simulink model "MCSI_simulation_2024_using_pc_source_and_cuantized_signals"  (R2021a)
settings: Solver=VariableStepAuto  StartTime=0.0  StopTime=10/cfg.fl  RelTol=1e-3
undefined symbols (not defined in the file or in its folder): cfg
libraries: spsIdealSwitchLib x18, simulink x8, spsSeriesRLCBranchLib x8, spsCurrentMeasurementLib x6, spsMosfetLib x4, commutil2 x3, spsTriangleGeneratorLib x3, spsMeanLib x2, spsThreePhaseSeriesRLCBranchLib x2, spsThreePhaseVIMeasurementLib x2, spspowerguiLib x2, spsGroundLib x1
settings Model: Creator=Damian  LastModifiedBy=Damian

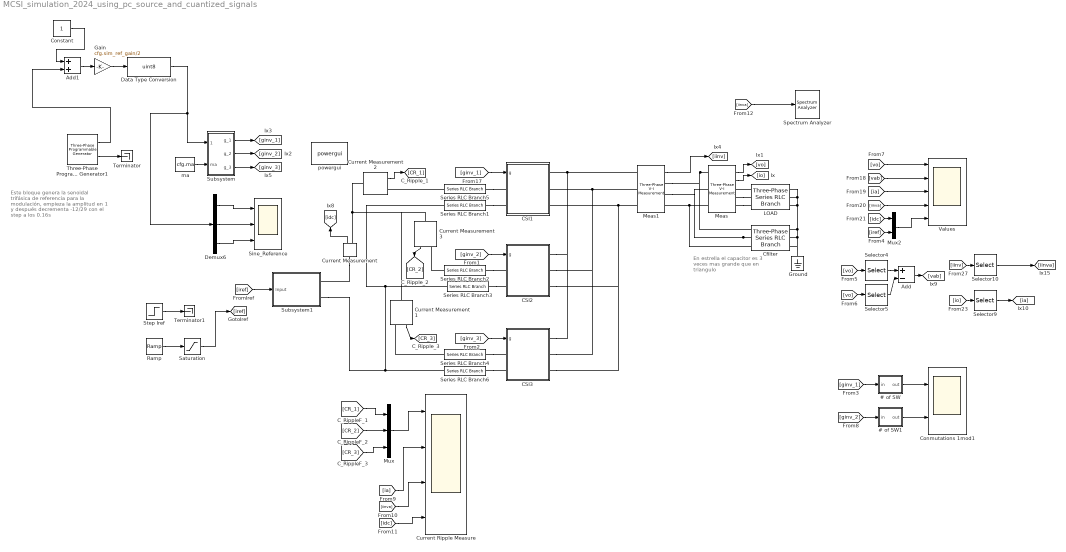
== system MCSI_simulation_2024_using_pc_source_and_cuantized_signals ==
  note: Este bloque genera la senoidal
      | trifásica de referencia para la
      | modulación, empieza la amplitud
      | en 1 y después decrementa -12/29
      | con el step a los 0.16s
  note: En estrella el capacitor
      | es 3 veces mas grande
      | que en triangulo
  # of SW : Subsystem
  # of SW1 : Subsystem
  Add : Sum  Inputs=+-
  Add1 : Sum
  CSI1 : Subsystem
  CSI2 : Subsystem
  CSI3 : Subsystem
  Cfilter : spsThreePhaseSeriesRLCBranchLib/Three-Phase Series RLC Branch  LConnTagsString=A|B|C  RConnTagsString=A|B|C  BranchType=C  Resistance=1  Inductance=cfg.c  Capacitance=cfg.c  Measurements=None
  Conmutations 1mod1 : Scope  NumInputPorts=2
  Constant : Constant
  Current Measurement{,1..3} (4 alike) : spsCurrentMeasurementLib/Current Measurement  PhasorSimulation=off  OutputType=Complex  PSBequivalent=0
  Current Ripple Measure : Scope  NumInputPorts=4
  Data Type Conversion : DataTypeConversion  OutDataTypeStr=uint8
  Demux6 : Demux  Outputs=3
  Gain : Gain  Gain=cfg.sim_ref_gain/2
  Ground : spsGroundLib/Ground  LConnTagsString=a
  LOAD : spsThreePhaseSeriesRLCBranchLib/Three-Phase Series RLC Branch  LConnTagsString=A|B|C  RConnTagsString=A|B|C  BranchType=RL  Resistance=cfg.r  Inductance=cfg.l  Capacitance=1e-6  Measurements=None
  Meas : spsThreePhaseVIMeasurementLib/Three-Phase V-I Measurement  VoltageMeasurement=phase-to-ground  SetLabelV=off  LabelV=Vabc  Vpu=off  VpuLL=off  CurrentMeasurement=yes  SetLabelI=off  LabelI=Iabc  Ipu=off  Pbase=100e6  Vbase=500e3  OutputType=Complex  PhasorSimulation=off  PSBequivalent=0
  Meas1 : spsThreePhaseVIMeasurementLib/Three-Phase V-I Measurement  VoltageMeasurement=no  SetLabelV=off  LabelV=Vabc  Vpu=off  VpuLL=off  CurrentMeasurement=yes  SetLabelI=off  LabelI=Iabc  Ipu=off  Pbase=100e6  Vbase=500e3  OutputType=Complex  PhasorSimulation=off  PSBequivalent=0
  Mux : Mux  Inputs=3
  Mux2 : Mux  Inputs=2
  Ramp : simulink/Sources/Ramp  slope=cfg.iref/cfg.cs_soft_start_time  start=0  InitialOutput=0
  Saturation : Saturate  UpperLimit=cfg.iref  LowerLimit=0
  Selector10 : Selector  InputPortWidth=3  IndexOptions=Index vector (dialog)  Indices=1  OutputSizes=1
  Selector4 : Selector  InputPortWidth=3  IndexOptions=Index vector (dialog)  Indices=1  OutputSizes=1
  Selector5 : Selector  InputPortWidth=3  IndexOptions=Index vector (dialog)  Indices=2  OutputSizes=1
  Selector9 : Selector  InputPortWidth=3  IndexOptions=Index vector (dialog)  Indices=1  OutputSizes=1
  Series RLC Branch{1..6} (6 alike) : spsSeriesRLCBranchLib/Series RLC Branch  LConnTagsString=__new0  RConnTagsString=__new0  BranchType=RL  Resistance=cfg.sharing_R  Inductance=cfg.sharing_L  SetiL0=off  InitialCurrent=0  Capacitance=1e-6  Setx0=off  InitialVoltage=0  Measurements=None
  Sine_Reference : Scope  NumInputPorts=3
  Spectrum Analyzer : SpectrumAnalyzer
  Step Iref : Step  Time=12/cfg.fl  Before=cfg.iref  After=0.6*cfg.iref  SampleTime=cfg.ts
  Subsystem : Subsystem
  Subsystem1 : Subsystem
  Terminator : Terminator
  Terminator1 : Terminator
  Three-Phase Programmable Generator1 : spsThreePhaseProgrammableGeneratorLib/Three-Phase Programmable Generator  Par_Vps=[0.9999,-30, cfg.fl]  VariationEntity=None  VariationType=Step  VariationStep=-12/29  VariationRate=10  VariationMag=0.3  VariationFreq=2  Par_Timing_Variation="[8/cfg.fl  10]"  SinglePhase=on  Yampli=[1 0.2 1.2 1.0]  Xtime=[0 0.1 0.15 0.2]  HarmonicGeneration=off  Par_HarmoA="[3  5  -25 0]"  Par_HarmoB="[5  10  35  2]"  Par_Timing_Harmo="[ 0.05  99]"  Ts=cfg.ts
      settings: SourceProductBaseCode=PS
  Values : Scope  NumInputPorts=5
  ma : Constant  Value=cfg.ma
  powergui : spspowerguiLib/powergui  Priority=1  SimulationMode=Discrete  SampleTime=cfg.ts  frequency=60  Iterations=50  frequencyindice=0  Pbase=100e6  ErrMax=1e-4  UnitsV=kV  UnitsW=MW  buscounter=0  FunctionMessages=off  echomessages=off  EnableUseOfTLC=off  CurrentSourceSwitches=off  DisableSnubberDevices=off  DisableRonSwitches=off  DisableVfSwitches=off  DisplayEquations=off  AutomaticDiscreteSolvers=off  SolverType=Backward Euler  Interpol=off  ExternalGateDelay=off  methode=off  Ts=0  x0status=blocks  SPID=off  SwTol=0  HookPort=off  NonlinearTolerance=1e-4  nMaxIteration=100  ContinueOnMaxIteration=off  RestoreLinks=warning  ResistiveCurrentMeasurement=off  Frange=[0:2:500]  Ylog=off  Xlog=on  ShowGrid=off  save=off  variable=ZData  structure=one_mod_model  ZoomFFT=off  StartTime=0.12  cycles=1  DisplayStyle=1  fundamental=50  FreqAxis=off  MaxFrequency=1000  frequencyindicesteady=1  RmsSteady=1  display=off
  wires:
  Current Measurement/1 -> [idc]
  ma/1 -> Subsystem/2(ma)
  Subsystem/1(g_1) -> [ginv_1]
  Three-Phase Programmable Generator1/2 -> Terminator/1
  Demux6/3 -> Sine_Reference/3
  Demux6/2 -> Sine_Reference/2
  Demux6/1 -> Sine_Reference/1
  [ginv_1] -> CSI1/1(g)
  Meas/1 -> [vo]
  Meas/2 -> [io]
  Meas1/1 -> [iinv]
  [iref] -> Mux2/2
  [idc] -> Mux2/1
  Mux2/1 -> Values/5
  [vo] -> Values/1
  [iinva] -> Values/4
  [ia] -> Values/3
  [vab] -> Values/2
  [vo] -> Selector4/1
  [vo] -> Selector5/1
  Selector4/1 -> Add/1
  Selector5/1 -> Add/2
  Add/1 -> [vab]
  [iinv] -> Selector10/1
  [io] -> Selector9/1
  Selector10/1 -> [iinva]
  Selector9/1 -> [ia]
  Subsystem/3(g_3) -> [ginv_3]
  Subsystem/2(g_2) -> [ginv_2]
  [ginv_2] -> CSI2/1(g)
  [ginv_3] -> CSI3/1(g)
  [ginv_1] -> # of SW/1(in)
  # of SW/1(out) -> Conmutations 1mod1/1
  # of SW1/1(out) -> Conmutations 1mod1/2
  [ginv_2] -> # of SW1/1(in)
  Saturation/1 -> [iref]
  Ramp/1 -> Saturation/1
  Step Iref/1 -> Terminator1/1
  Current Measurement2/1 -> [CR_1]
  Current Measurement3/1 -> [CR_2]
  Current Measurement1/1 -> [CR_3]
  [ia] -> Current Ripple Measure/2
  [iinva] -> Current Ripple Measure/3
  [idc] -> Current Ripple Measure/4
  [CR_1] -> Mux/1
  [CR_2] -> Mux/2
  [CR_3] -> Mux/3
  Mux/1 -> Current Ripple Measure/1
  [iref] -> Subsystem1/1(Input)
  Constant/1 -> Add1/1
  Gain/1 -> Data Type Conversion/1
  Add1/1 -> Gain/1
  Three-Phase Programmable Generator1/1 -> Add1/2
  Data Type Conversion/1 -> Demux6/1, Subsystem/1(Vabc)
  [iinva] -> Spectrum Analyzer/1
  connections:
  Current Measurement/LConn1 -- Subsystem1/RConn1
  Meas/LConn3 -- Cfilter/LConn3 -- Meas1/RConn3
  Meas/LConn1 -- Meas1/RConn1 -- Cfilter/LConn1
  LOAD/RConn2 -- LOAD/RConn1 -- LOAD/RConn3 -- Cfilter/RConn1 -- Cfilter/RConn2 -- Cfilter/RConn3 -- Ground/LConn1
  Cfilter/LConn2 -- Meas1/RConn2 -- Meas/LConn2
  LOAD/LConn1 -- Meas/RConn1
  Meas/RConn2 -- LOAD/LConn2
  Meas/RConn3 -- LOAD/LConn3
  Meas1/LConn1 -- CSI3/RConn1 -- CSI2/RConn1 -- CSI1/RConn1
  Meas1/LConn2 -- CSI3/RConn2 -- CSI2/RConn2 -- CSI1/RConn2
  Meas1/LConn3 -- CSI3/RConn3 -- CSI2/RConn3 -- CSI1/RConn3
  Series RLC Branch1/RConn1 -- CSI1/LConn2
  Series RLC Branch5/RConn1 -- CSI1/LConn1
  Series RLC Branch2/RConn1 -- CSI2/LConn1
  Series RLC Branch3/RConn1 -- CSI2/LConn2
  Series RLC Branch4/RConn1 -- CSI3/LConn1
  Series RLC Branch6/RConn1 -- CSI3/LConn2
  Subsystem1/RConn2 -- Series RLC Branch6/LConn1 -- Series RLC Branch3/LConn1 -- Series RLC Branch1/LConn1
  Series RLC Branch2/LConn1 -- Current Measurement3/RConn1
  Current Measurement2/LConn1 -- Current Measurement3/LConn1 -- Current Measurement1/LConn1 -- Current Measurement/RConn1
  Series RLC Branch4/LConn1 -- Current Measurement1/RConn1
  Series RLC Branch5/LConn1 -- Current Measurement2/RConn1

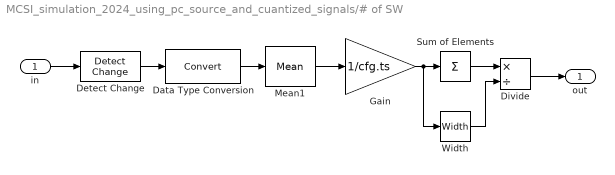
== system MCSI_simulation_2024_using_pc_source_and_cuantized_signals/# of SW ==
  in : Inport
  Data Type Conversion : DataTypeConversion
  Detect Change : simulink/Logic and Bit Operations/Detect Change  vinit=0  OutDataTypeStr=boolean
  Divide : Product  Inputs=*/
  Gain : Gain  Gain=1/cfg.ts
  Mean1 : spsMeanLib/Mean  Freq=cfg.fl  Vinit=0  Ts=cfg.ts
  Sum of Elements : Sum  Inputs=+
  Width : Width
  out : Outport
  wires:
  Detect Change/1 -> Data Type Conversion/1
  Mean1/1 -> Gain/1
  Data Type Conversion/1 -> Mean1/1
  in/1 -> Detect Change/1
  Gain/1 -> Width/1, Sum of Elements/1
  Sum of Elements/1 -> Divide/1
  Width/1 -> Divide/2
  Divide/1 -> out/1

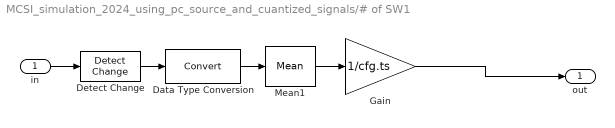
== system MCSI_simulation_2024_using_pc_source_and_cuantized_signals/# of SW1 ==
  in : Inport
  Data Type Conversion : DataTypeConversion
  Detect Change : simulink/Logic and Bit Operations/Detect Change  vinit=0  OutDataTypeStr=boolean
  Gain : Gain  Gain=1/cfg.ts
  Mean1 : spsMeanLib/Mean  Freq=cfg.fl  Vinit=0  Ts=cfg.ts
  out : Outport
  wires:
  Detect Change/1 -> Data Type Conversion/1
  Mean1/1 -> Gain/1
  Data Type Conversion/1 -> Mean1/1
  in/1 -> Detect Change/1
  Gain/1 -> out/1

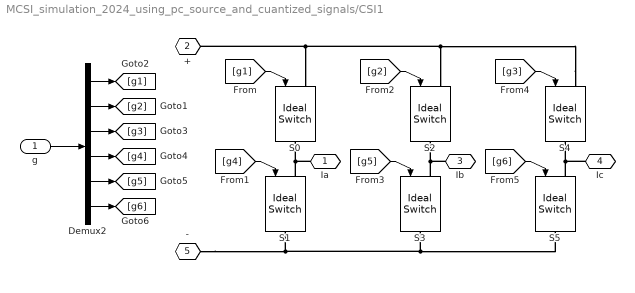
== system MCSI_simulation_2024_using_pc_source_and_cuantized_signals/CSI1 ==
  g : Inport
  Demux2 : Demux  Outputs=6
  S{0..5} (6 alike) : spsIdealSwitchLib/Ideal Switch  Ron=cfg.switch.Ron  Lon=0  IC=0  Rs=cfg.switch.snubber_Rs  Cs=cfg.switch.snubber_Cs  Measurements=off
  Ia : PMIOPort  Side=Right
  + : PMIOPort  Port=2  Side=Left
  Ib : PMIOPort  Port=3  Side=Right
  Ic : PMIOPort  Port=4  Side=Right
  - : PMIOPort  Port=5  Side=Left
  wires:
  Demux2/1 -> [g1]
  Demux2/4 -> [g4]
  g/1 -> Demux2/1
  [g4] -> S1/1
  [g2] -> S2/1
  [g5] -> S3/1
  Demux2/5 -> [g5]
  [g3] -> S4/1
  [g6] -> S5/1
  Demux2/6 -> [g6]
  Demux2/3 -> [g3]
  Demux2/2 -> [g2]
  [g1] -> S0/1
  connections:
  S1/LConn1 -- Ia/RConn1 -- S0/RConn1
  S3/LConn1 -- Ib/RConn1 -- S2/RConn1
  S5/LConn1 -- Ic/RConn1 -- S4/RConn1
  S4/LConn1 -- S2/LConn1 -- S0/LConn1 -- +/RConn1
  -/RConn1 -- S5/RConn1 -- S3/RConn1 -- S1/RConn1

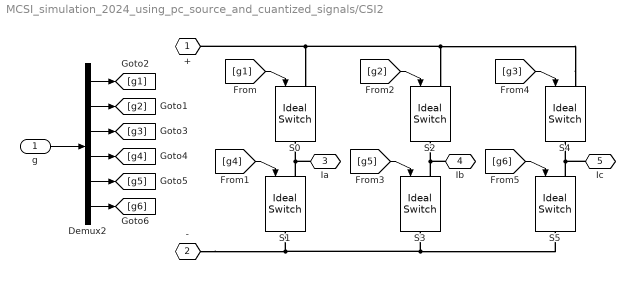
== system MCSI_simulation_2024_using_pc_source_and_cuantized_signals/CSI2 ==
  g : Inport
  Demux2 : Demux  Outputs=6
  S{0..5} (6 alike) : spsIdealSwitchLib/Ideal Switch  Ron=cfg.switch.Ron  Lon=0  IC=0  Rs=cfg.switch.snubber_Rs  Cs=cfg.switch.snubber_Cs  Measurements=off
  + : PMIOPort  Side=Left
  - : PMIOPort  Port=2  Side=Left
  Ia : PMIOPort  Port=3  Side=Right
  Ib : PMIOPort  Port=4  Side=Right
  Ic : PMIOPort  Port=5  Side=Right
  wires:
  Demux2/1 -> [g1]
  Demux2/4 -> [g4]
  g/1 -> Demux2/1
  [g4] -> S1/1
  [g2] -> S2/1
  [g5] -> S3/1
  Demux2/5 -> [g5]
  [g3] -> S4/1
  [g6] -> S5/1
  Demux2/6 -> [g6]
  Demux2/3 -> [g3]
  Demux2/2 -> [g2]
  [g1] -> S0/1
  connections:
  S1/LConn1 -- Ia/RConn1 -- S0/RConn1
  S3/LConn1 -- Ib/RConn1 -- S2/RConn1
  S5/LConn1 -- Ic/RConn1 -- S4/RConn1
  S4/LConn1 -- S2/LConn1 -- S0/LConn1 -- +/RConn1
  -/RConn1 -- S5/RConn1 -- S3/RConn1 -- S1/RConn1

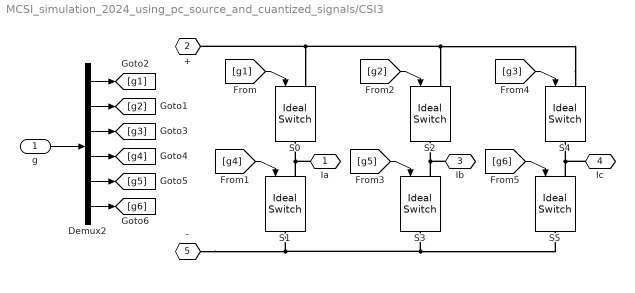
== system MCSI_simulation_2024_using_pc_source_and_cuantized_signals/CSI3 ==
  g : Inport
  Demux2 : Demux  Outputs=6
  S{0..5} (6 alike) : spsIdealSwitchLib/Ideal Switch  Ron=cfg.switch.Ron  Lon=0  IC=0  Rs=cfg.switch.snubber_Rs  Cs=cfg.switch.snubber_Cs  Measurements=off
  Ia : PMIOPort  Side=Right
  + : PMIOPort  Port=2  Side=Left
  Ib : PMIOPort  Port=3  Side=Right
  Ic : PMIOPort  Port=4  Side=Right
  - : PMIOPort  Port=5  Side=Left
  wires:
  Demux2/1 -> [g1]
  Demux2/4 -> [g4]
  g/1 -> Demux2/1
  [g4] -> S1/1
  [g2] -> S2/1
  [g5] -> S3/1
  Demux2/5 -> [g5]
  [g3] -> S4/1
  [g6] -> S5/1
  Demux2/6 -> [g6]
  Demux2/3 -> [g3]
  Demux2/2 -> [g2]
  [g1] -> S0/1
  connections:
  S1/LConn1 -- Ia/RConn1 -- S0/RConn1
  S3/LConn1 -- Ib/RConn1 -- S2/RConn1
  S5/LConn1 -- Ic/RConn1 -- S4/RConn1
  S4/LConn1 -- S2/LConn1 -- S0/LConn1 -- +/RConn1
  -/RConn1 -- S5/RConn1 -- S3/RConn1 -- S1/RConn1

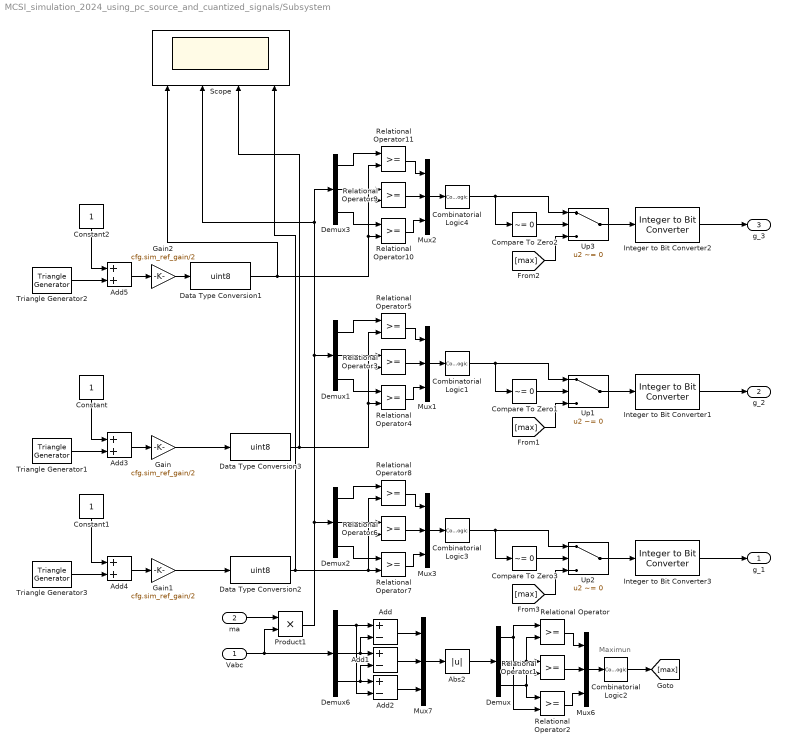
== system MCSI_simulation_2024_using_pc_source_and_cuantized_signals/Subsystem ==
  note: Maximun
  Vabc : Inport
  ma : Inport  Port=2
  Abs2 : Abs
  Add : Sum  Inputs=+-
  Add1 : Sum  Inputs=+-
  Add2 : Sum  Inputs=+-
  Add3 : Sum
  Add4 : Sum
  Add5 : Sum
  Combinatorial Logic1 : CombinatorialLogic  TruthTable=bin2dec(['000000'; '001010'; '010100'; '001100'; '100001'; '100010'; '010001'; '000000'])
  Combinatorial Logic2 : CombinatorialLogic  TruthTable=bin2dec(['111111'; '001001'; '010010'; '010010'; '100100'; '001001'; '100100'; '111111'])
  Combinatorial Logic3 : CombinatorialLogic  TruthTable=bin2dec(['000000'; '001010'; '010100'; '001100'; '100001'; '100010'; '010001'; '000000'])
  Combinatorial Logic4 : CombinatorialLogic  TruthTable=bin2dec(['000000'; '001010'; '010100'; '001100'; '100001'; '100010'; '010001'; '000000'])
  Compare To Zero1 : simulink/Logic and Bit Operations/Compare To Zero  relop=~=  OutDataTypeStr=boolean
  Compare To Zero2 : simulink/Logic and Bit Operations/Compare To Zero  relop=~=  OutDataTypeStr=boolean
  Compare To Zero3 : simulink/Logic and Bit Operations/Compare To Zero  relop=~=  OutDataTypeStr=boolean
  Constant : Constant
  Constant1 : Constant
  Constant2 : Constant
  Data Type Conversion1 : DataTypeConversion  OutDataTypeStr=uint8
  Data Type Conversion2 : DataTypeConversion  OutDataTypeStr=uint8
  Data Type Conversion3 : DataTypeConversion  OutDataTypeStr=uint8
  Demux{,1..3,6} (5 alike) : Demux  Outputs=3
  Gain : Gain  Gain=cfg.sim_ref_gain/2
  Gain1 : Gain  Gain=cfg.sim_ref_gain/2
  Gain2 : Gain  Gain=cfg.sim_ref_gain/2
  Integer to Bit Converter1 : commutil2/Integer to Bit Converter  nbits=6  signedInputValues=Unsigned  bitOrder=MSB first  outDtype=Inherit via internal rule
  Integer to Bit Converter2 : commutil2/Integer to Bit Converter  nbits=6  signedInputValues=Unsigned  bitOrder=MSB first  outDtype=Inherit via internal rule
  Integer to Bit Converter3 : commutil2/Integer to Bit Converter  nbits=6  signedInputValues=Unsigned  bitOrder=MSB first  outDtype=Inherit via internal rule
  Mux{1..3,6..7} (5 alike) : Mux  Inputs=3
  Product1 : Product
  Relational Operator{,1..11} (12 alike) : RelationalOperator  OutDataTypeStr=boolean  RndMeth=Nearest
  Scope : Scope  NumInputPorts=4
  Triangle Generator1 : spsTriangleGeneratorLib/Triangle Generator  Freq=cfg.fl*cfg.mf  Phase=120  Ts=cfg.ts
  Triangle Generator2 : spsTriangleGeneratorLib/Triangle Generator  Freq=cfg.fl*cfg.mf  Phase=240  Ts=cfg.ts
  Triangle Generator3 : spsTriangleGeneratorLib/Triangle Generator  Freq=cfg.fl*cfg.mf  Phase=0  Ts=cfg.ts
  Up1 : Switch  Criteria=u2 ~= 0
  Up2 : Switch  Criteria=u2 ~= 0
  Up3 : Switch  Criteria=u2 ~= 0
  g_1 : Outport
  g_2 : Outport  Port=2
  g_3 : Outport  Port=3
  wires:
  Relational Operator/1 -> Mux6/1
  Demux/3 -> Relational Operator1/2, Relational Operator2/1
  Relational Operator1/1 -> Mux6/2
  Demux/2 -> Relational Operator/2, Relational Operator1/1
  Mux6/1 -> Combinatorial Logic2/1
  Relational Operator2/1 -> Mux6/3
  Vabc/1 -> Product1/2, Demux6/1
  Demux/1 -> Relational Operator/1, Relational Operator2/2
  Demux6/1 -> Add2/2, Add/1
  Demux6/2 -> Add/2, Add1/1
  Demux6/3 -> Add1/2, Add2/1
  Add/1 -> Mux7/1
  Add1/1 -> Mux7/2
  Add2/1 -> Mux7/3
  Abs2/1 -> Demux/1
  Mux7/1 -> Abs2/1
  Combinatorial Logic2/1 -> [max]
  ma/1 -> Product1/1
  Relational Operator7/1 -> Mux3/3
  Relational Operator8/1 -> Mux3/1
  Relational Operator6/1 -> Mux3/2
  Mux3/1 -> Combinatorial Logic3/1
  Combinatorial Logic3/1 -> Up2/1, Compare To Zero3/1
  Compare To Zero3/1 -> Up2/2
  Up2/1 -> Integer to Bit Converter3/1
  [max] -> Up2/3
  Demux2/3 -> Relational Operator7/1
  Demux2/2 -> Relational Operator6/1
  Demux2/1 -> Relational Operator8/1
  Integer to Bit Converter3/1 -> g_1/1
  Integer to Bit Converter1/1 -> g_2/1
  Relational Operator5/1 -> Mux1/1
  Demux1/1 -> Relational Operator5/1
  Mux1/1 -> Combinatorial Logic1/1
  Relational Operator3/1 -> Mux1/2
  [max] -> Up1/3
  Combinatorial Logic1/1 -> Up1/1, Compare To Zero1/1
  Demux1/2 -> Relational Operator3/1
  Up1/1 -> Integer to Bit Converter1/1
  Demux1/3 -> Relational Operator4/1
  Relational Operator4/1 -> Mux1/3
  Compare To Zero1/1 -> Up1/2
  Compare To Zero2/1 -> Up3/2
  Up3/1 -> Integer to Bit Converter2/1
  Relational Operator10/1 -> Mux2/3
  Demux3/2 -> Relational Operator9/1
  Demux3/3 -> Relational Operator10/1
  Relational Operator9/1 -> Mux2/2
  [max] -> Up3/3
  Demux3/1 -> Relational Operator11/1
  Combinatorial Logic4/1 -> Up3/1, Compare To Zero2/1
  Integer to Bit Converter2/1 -> g_3/1
  Relational Operator11/1 -> Mux2/1
  Mux2/1 -> Combinatorial Logic4/1
  Product1/1 -> Scope/2, Demux3/1, Demux1/1, Demux2/1
  Data Type Conversion3/1 -> Scope/3, Relational Operator5/2, Relational Operator3/2, Relational Operator4/2
  Data Type Conversion1/1 -> Scope/1, Relational Operator11/2, Relational Operator9/2, Relational Operator10/2
  Data Type Conversion2/1 -> Relational Operator8/2, Relational Operator6/2, Relational Operator7/2, Scope/4
  Gain/1 -> Data Type Conversion3/1
  Gain1/1 -> Data Type Conversion2/1
  Gain2/1 -> Data Type Conversion1/1
  Triangle Generator1/1 -> Add3/2
  Add3/1 -> Gain/1
  Constant/1 -> Add3/1
  Constant1/1 -> Add4/1
  Triangle Generator3/1 -> Add4/2
  Add4/1 -> Gain1/1
  Add5/1 -> Gain2/1
  Constant2/1 -> Add5/1
  Triangle Generator2/1 -> Add5/2

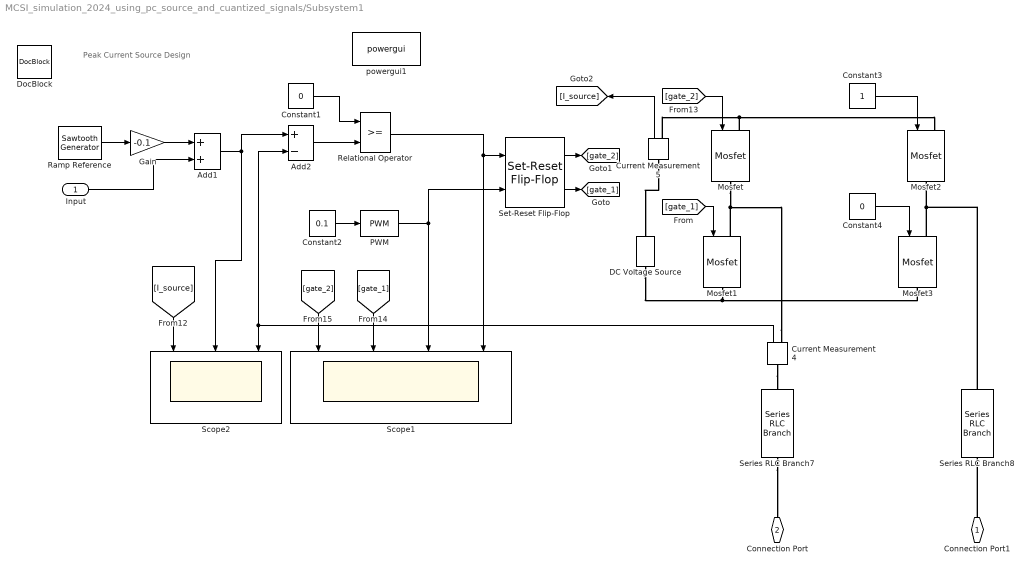
== system MCSI_simulation_2024_using_pc_source_and_cuantized_signals/Subsystem1 ==
  note: Peak Current Source Design
  Input : Inport
  Add1 : Sum
  Add2 : Sum  Inputs=+-
  Constant1 : Constant  Value=0
  Constant2 : Constant  Value=0.1
  Constant3 : Constant
  Constant4 : Constant  Value=0
  Current Measurement4 : spsCurrentMeasurementLib/Current Measurement  PhasorSimulation=off  OutputType=Complex  PSBequivalent=0
  Current Measurement5 : spsCurrentMeasurementLib/Current Measurement  PhasorSimulation=off  OutputType=Complex  PSBequivalent=0
  DC Voltage Source : spsDCVoltageSourceLib/DC Voltage Source  Amplitude=100  Measurements=None
  DocBlock : simulink/Model-Wide Utilities/DocBlock  DocumentType=Text
      content=|
      | Ramp is added to reference to avoid subharmonic oscilations.
      |
      | Check NxP AN4716: https://www.nxp.com/docs/en/application-note/AN4716.pdf
  Gain : Gain  Gain=-0.1
  Mosfet{,1..3} (4 alike) : spsMosfetLib/Mosfet  Ron=0.1  Lon=0  Rd=0.01  Vfd=0  IC=0  Rs=1e5  Cs=inf  Measurements=off
  PWM : simulink/Discontinuities/PWM  DisableCoverage=on  Period=1E-5  DisallowZeroDutyCycle=off  RunAtFixedTimeIntervals=off  SampleTime=0.1
  Ramp Reference : spsSawtoothGeneratorLib/Sawtooth Generator  Freq=10e3  Phase=0  Ts=0
  Relational Operator : RelationalOperator  OutDataTypeStr=boolean  RndMeth=Simplest
  Scope1 : Scope  NumInputPorts=4
  Scope2 : Scope  NumInputPorts=3
  Series RLC Branch7 : spsSeriesRLCBranchLib/Series RLC Branch  LConnTagsString=__new0  RConnTagsString=__new0  BranchType=L  Resistance=1  Inductance=cfg.main_L  SetiL0=off  InitialCurrent=0  Capacitance=1e-6  Setx0=off  InitialVoltage=0  Measurements=Branch current
  Series RLC Branch8 : spsSeriesRLCBranchLib/Series RLC Branch  LConnTagsString=__new0  RConnTagsString=__new0  BranchType=L  Resistance=1  Inductance=cfg.main_L  SetiL0=off  InitialCurrent=0  Capacitance=1e-6  Setx0=off  InitialVoltage=0  Measurements=Branch current
  Set-Reset Flip-Flop : eeGeneralControl/Set-Reset Flip-Flop  LabelModeActiveChoice=Discrete  UndefState=Reset  Q0=0  Ts=-1
      settings: SourceProductBaseCode=PS
  powergui1 : spspowerguiLib/powergui  Priority=1  SimulationMode=Discrete  SampleTime=1e-8  frequency=60  Iterations=50  frequencyindice=0  Pbase=100e6  ErrMax=1e-4  UnitsV=kV  UnitsW=MW  buscounter=0  FunctionMessages=off  echomessages=off  EnableUseOfTLC=off  CurrentSourceSwitches=off  DisableSnubberDevices=off  DisableRonSwitches=off  DisableVfSwitches=off  DisplayEquations=off  AutomaticDiscreteSolvers=off  SolverType=Tustin/Backward Euler (TBE)  Interpol=off  ExternalGateDelay=off  methode=off  Ts=100  x0status=blocks  SPID=on  SwTol=0  HookPort=off  NonlinearTolerance=1e-4  nMaxIteration=100  ContinueOnMaxIteration=off  RestoreLinks=warning  ResistiveCurrentMeasurement=off  Frange=[0:2:500]  Ylog=off  Xlog=on  ShowGrid=off  save=off  variable=ZData  structure=0  ZoomFFT=off  StartTime=0.0  cycles=1  DisplayStyle=1  fundamental=60  FreqAxis=off  MaxFrequency=1000  frequencyindicesteady=1  RmsSteady=1  display=off
  Connection Port1 : PMIOPort  Side=Right
  Connection Port : PMIOPort  Port=2  Side=Right
  wires:
  Current Measurement5/1 -> [I_source]
  [gate_2] -> Mosfet/1
  Current Measurement4/1 -> Scope2/3, Add2/2
  PWM/1 -> Set-Reset Flip-Flop/2, Scope1/3
  Set-Reset Flip-Flop/1 -> [gate_2]
  Ramp Reference/1 -> Gain/1
  [gate_1] -> Scope1/2
  [I_source] -> Scope2/1
  Constant4/1 -> Mosfet3/1
  Add2/1 -> Relational Operator/2
  Constant2/1 -> PWM/1
  Constant3/1 -> Mosfet2/1
  Add1/1 -> Scope2/2, Add2/1
  [gate_1] -> Mosfet1/1
  Gain/1 -> Add1/1
  Input/1 -> Add1/2
  [gate_2] -> Scope1/1
  Set-Reset Flip-Flop/2 -> [gate_1]
  Relational Operator/1 -> Set-Reset Flip-Flop/1, Scope1/4
  Constant1/1 -> Relational Operator/1
  connections:
  Mosfet2/LConn1 -- Mosfet/LConn1 -- Current Measurement5/RConn1
  Series RLC Branch7/RConn1 -- Connection Port/RConn1
  Mosfet3/RConn1 -- Mosfet1/RConn1 -- DC Voltage Source/LConn1
  Current Measurement4/LConn1 -- Series RLC Branch7/LConn1
  Connection Port1/RConn1 -- Series RLC Branch8/RConn1
  Current Measurement5/LConn1 -- DC Voltage Source/RConn1
  Current Measurement4/RConn1 -- Mosfet1/LConn1 -- Mosfet/RConn1
  Mosfet2/RConn1 -- Series RLC Branch8/LConn1 -- Mosfet3/LConn1
